simulink model "logic111"  (Simulink 8.8)
settings: Solver=VariableStepAuto  StartTime=0.0  StopTime=10.0  RelTol=1e-3
libraries: simulink x5
settings Model: Creator=viett  LastModifiedBy=viett
settings DataIOCC: LimitDataPoints=off  SaveFormat=Dataset  SignalLoggingSaveFormat=Dataset
settings OptimizationCC: LifeSpan=auto
settings DebuggingCC: UnderspecifiedInitializationDetection=Simplified  MergeDetectMultiDrivingBlocksExec=error  FcnCallInpInsideContextMsg=error  StateNameClashWarn=none  SFUnexpectedBacktrackingDiag=error  SFNoUnconditionalDefaultTransitionDiag=error  SFExecutionAtInitializationDiag=warning
settings HardwareCC: ProdBitPerPointer=64  ProdBitPerSizeT=64  ProdBitPerPtrDiffT=64  ProdLargestAtomicFloat=Float  ProdIntDivRoundTo=Zero  ProdEndianess=LittleEndian  ProdWordSize=64  ProdHWDeviceType=Intel->x86-64 (Windows64)
settings ModelReferenceCC: PropagateSignalLabelsOutOfModel=on
settings GRTTargetCC: TargetLangStandard=C99 (ISO)  GeneratePreprocessorConditionals=Use local settings  CombineOutputUpdateFcns=on  GRTInterface=off
settings ConfigComp: CovMetricSettings=dwe  CovHtmlReporting=off  CovSaveCumulativeToWorkspaceVar=off  CovSaveSingleToWorkspaceVar=off  CovExternalEMLEnable=on

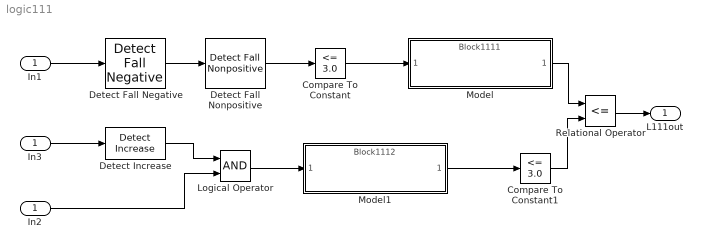
== system logic111 ==
  In1 : Inport
  Compare To Constant : simulink/Logic and Bit Operations/Compare To Constant  relop=<=  const=3.0  OutDataTypeStr=boolean
  Compare To Constant1 : simulink/Logic and Bit Operations/Compare To Constant  relop=<=  const=3.0  OutDataTypeStr=boolean
  Detect Increase : simulink/Logic and Bit Operations/Detect Increase  vinit=0.0  OutDataTypeStr=boolean
  Detect Fall Negative : simulink/Logic and Bit Operations/Detect Fall Negative  vinit=0  OutDataTypeStr=boolean
  Detect Fall Nonpositive : simulink/Logic and Bit Operations/Detect Fall Nonpositive  vinit=0  OutDataTypeStr=boolean
  In2 : InportShadow
  In3 : InportShadow
  Logical Operator : Logic  AllPortsSameDT=off  OutDataTypeStr=boolean
  Model : ModelReference  ModelNameDialog=Block1111.slx  SimulationMode=Normal  ModelReferenceVersion=1.4
  Model1 : ModelReference  ModelNameDialog=Block1112  SimulationMode=Normal  ModelReferenceVersion=1.1
  Relational Operator : RelationalOperator  Operator=<=  OutDataTypeStr=boolean  RndMeth=Simplest
  L111out : Outport
  wires:
  Detect Fall Negative/1 -> Detect Fall Nonpositive/1
  Detect Fall Nonpositive/1 -> Compare To Constant/1
  Compare To Constant/1 -> Model/1
  In1/1 -> Detect Fall Negative/1
  Model/1 -> Relational Operator/1
  Model1/1 -> Compare To Constant1/1
  In2/1 -> Logical Operator/2
  Compare To Constant1/1 -> Relational Operator/2
  Logical Operator/1 -> Model1/1
  Detect Increase/1 -> Logical Operator/1
  In3/1 -> Detect Increase/1
  Relational Operator/1 -> L111out/1
